simulink model "LQR_Lateral_Stability"  (R2019a)
settings: Solver=FixedStepAuto  StartTime=0.0  StopTime=10.0  FixedStep=0.1  RelTol=1e-3
values from neighbouring files (symbols this model uses):
  A = [-(Cf+Cr)/(m*Vx), -1-(lf*Cf-lr*Cr)/(m*Vx^2) ... (first row only)    [LQI_for_LateralStability_LinMod_slipNDyaw.m]    (also in LQR.m; LQR_Model_Initialization.m; LQR_Simulink_testData_DLC.mat = [-4.40211640212  -0.830687830688; 20.8695652174  -5.18678260; LQR_test_data_DLC.mat = [-4.40211640212  -0.830687830688; 20.8695652174  -5.18678260)
  B = [Cf/(m*Vx);(lf*Cf)/Iz]    [LQI_for_LateralStability_LinMod_slipNDyaw.m]    (also in LQR.m; LQR_Model_Initialization.m; LQR_Simulink_testData_DLC.mat = [1.60846560847 15.8608695652]; LQR_test_data_DLC.mat = [1.60846560847 15.8608695652])
  Kc_lqi_t1 = lqi(ss(A,B,C_lqi,D),Q_lqi,R_lqi)    [LQI_for_LateralStability_LinMod_slipNDyaw.m]    (also in LQR_Simulink_testData_DLC.mat = [1.01738471556 0.836422769782 0.0467371713947 -9.99890775876)
settings Model: Creator=Shouvik Chakraborty  LastModifiedBy=Shouvik Chakraborty
settings DataIOCC: ReturnWorkspaceOutputs=off
settings DebuggingCC: PregeneratedLibrarySubsystemCodeDiagnostic=none  ArithmeticOperatorsInVariantConditions=warning
settings SFSimCC: SimUseLocalCustomCode=off
settings RTWCC: RTWUseLocalCustomCode=off

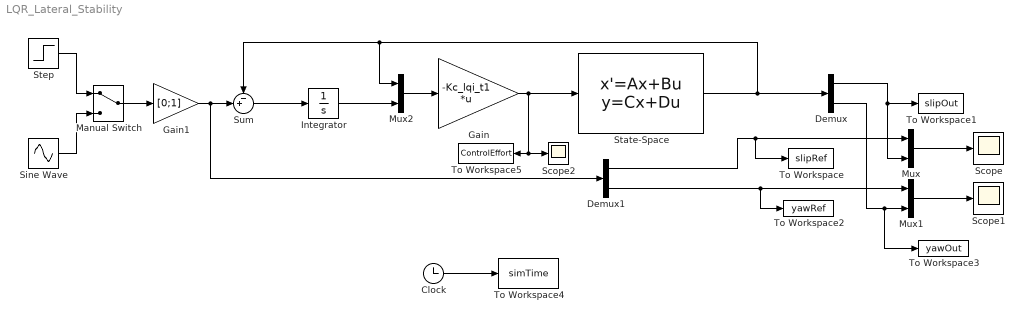
== system LQR_Lateral_Stability ==
  Clock : Clock
  Demux : Demux  Outputs=2
  Demux1 : Demux  Outputs=2
  Gain : Gain  Gain=-Kc_lqi_t1  Multiplication=Matrix(K*u)
  Gain1 : Gain  Gain=[0;1]
  Integrator : Integrator
  Manual Switch : ManualSwitch
  Mux : Mux  Inputs=2
  Mux1 : Mux  Inputs=2
  Mux2 : Mux  Inputs=2
  Scope : Scope
  Scope1 : Scope
  Scope2 : Scope
  Sine Wave : Sin  Amplitude=2  Frequency=0.5  SampleTime=0
  State-Space : StateSpace  A=A  B=B  C=eye(2,2)  D=[0;0]  InitialCondition=0
  Step : Step  SampleTime=0
  Sum : Sum  Inputs=-+|
  To Workspace : ToWorkspace  VariableName=slipRef  SampleTime=-1
  To Workspace1 : ToWorkspace  VariableName=slipOut  SampleTime=-1
  To Workspace2 : ToWorkspace  VariableName=yawRef  SampleTime=-1
  To Workspace3 : ToWorkspace  VariableName=yawOut  SampleTime=-1
  To Workspace4 : ToWorkspace  VariableName=simTime  SampleTime=-1
  To Workspace5 : ToWorkspace  VariableName=ControlEffort  SampleTime=-1
  wires:
  State-Space/1 -> Sum/1, Mux2/1, Demux/1
  Mux2/1 -> Gain/1
  Integrator/1 -> Mux2/2
  Sum/1 -> Integrator/1
  Gain1/1 -> Demux1/1, Sum/2
  Manual Switch/1 -> Gain1/1
  Sine Wave/1 -> Manual Switch/2
  Step/1 -> Manual Switch/1
  Demux/1 -> To Workspace1/1, Mux/2
  Demux/2 -> To Workspace3/1, Mux1/2
  Demux1/1 -> To Workspace/1, Mux/1
  Demux1/2 -> To Workspace2/1, Mux1/1
  Mux/1 -> Scope/1
  Mux1/1 -> Scope1/1
  Gain/1 -> State-Space/1, Scope2/1, To Workspace5/1
  Clock/1 -> To Workspace4/1
